simulink library "iq_mixer_8c4r_lib"  (Simulink 8.7)
settings: Solver=ode45  StartTime=0.0  StopTime=10.0  RelTol=1e-3
undefined symbols (not defined in the file): AdvDSPBChannelOutDisplay, dpoly, dspba_ChannelInVis, dspba_ChannelOutVis, dspba_internal_get_channel_ports, dspba_internal_get_demux_ports, evalAionMaskParam, latency, primtype, value
libraries: DSPBAPrim x25, Pipereg_lib x2, DSPBABase x1
settings Model: Creator=bigcat  LastModifiedBy=5g

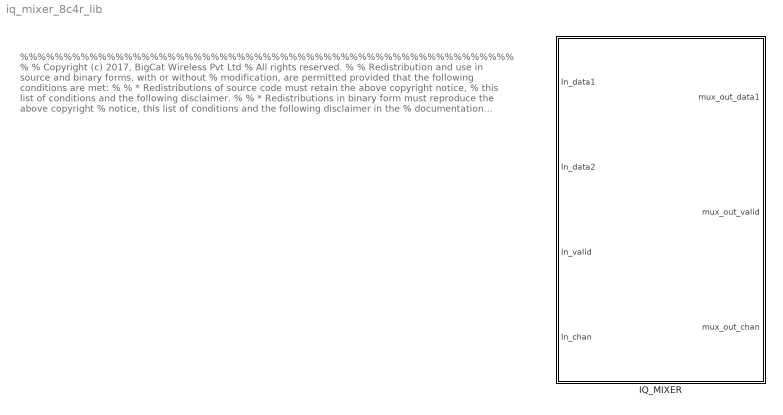
== system iq_mixer_8c4r_lib ==
  note: %%%%%%%%%%%%%%%%%%%%%%%%%%%%%%%%%%%%%%%%%%%%%%%%%%%%%%%%%
      |  %
      |  % Copyright (c) 2017, BigCat Wireless Pvt Ltd
      |  % All rights reserved.
      |  %
      |  % Redistribution and use in source and binary forms, with or without
      |  % modification, are permitted provided that the following conditions are met:
      |  %
      |  %     * Redistributions of source code must retain the above copyright notice,
      |  %       this list of conditions and the following disclaimer.
      |  %
      |  %     * Redistributions in binary form must reproduce the above copyright
      |  %       notice, this list of conditions and the following disclaimer in the
      |  %       documentation and/or other materials provided with the distribution.
      |  %
      |  %     * Neither the name of the copyright holder nor the names of its contributors
      |  %       may be used to endorse or promote products derived from this software
      |  %       without specific prior written permission.
      |  %
      |  %
      |  %
      |  % THIS SOFTWARE IS PROVIDED BY THE COPYRIGHT HOLDERS AND CONTRIBUTORS "AS IS"
      |  % AND ANY EXPRESS OR IMPLIED WARRANTIES, INCLUDING, BUT NOT LIMITED TO, THE
      |  % IMPLIED WARRANTIES OF MERCHANTABILITY AND FITNESS FOR A PARTICULAR PURPOSE ARE
      |  % DISCLAIMED. IN NO EVENT SHALL THE COPYRIGHT HOLDER OR CONTRIBUTORS BE LIABLE
      |  % FOR ANY DIRECT, INDIRECT, INCIDENTAL, SPECIAL, EXEMPLARY, OR CONSEQUENTIAL
      |  % DAMAGES (INCLUDING, BUT NOT LIMITED TO, PROCUREMENT OF SUBSTITUTE GOODS OR
      |  % SERVICES; LOSS OF USE, DATA, OR PROFITS; OR BUSINESS INTERRUPTION) HOWEVER
      |  % CAUSED AND ON ANY THEORY OF LIABILITY, WHETHER IN CONTRACT, STRICT LIABILITY,
      |  % OR TORT (INCLUDING NEGLIGENCE OR OTHERWISE) ARISING IN ANY WAY OUT OF THE USE
      |  % OF THIS SOFTWARE, EVEN IF ADVISED OF THE POSSIBILITY OF SUCH DAMAGE.
      |  %
      |   %%%%%%%%%%%%%%%%%%%%%%%%%%%%%%%%%%%%%%%%%%%%%%%%%%%%%%%%%%
  IQ_MIXER : Subsystem  mask{Latency=0, ClockMargin=0, Pipeline_stages=0}
      mask Display:
      | disp('IQ_MIXER');
      | port_label('input',1,'d_I');
      | port_label('input',2,'d_Q');
      | port_label('input',3,'v');
      | port_label('input',4,'c');
      | port_label('output',1,'q');
      | port_label('output',2,'q_v');
      | port_label('output',3,'q_c');

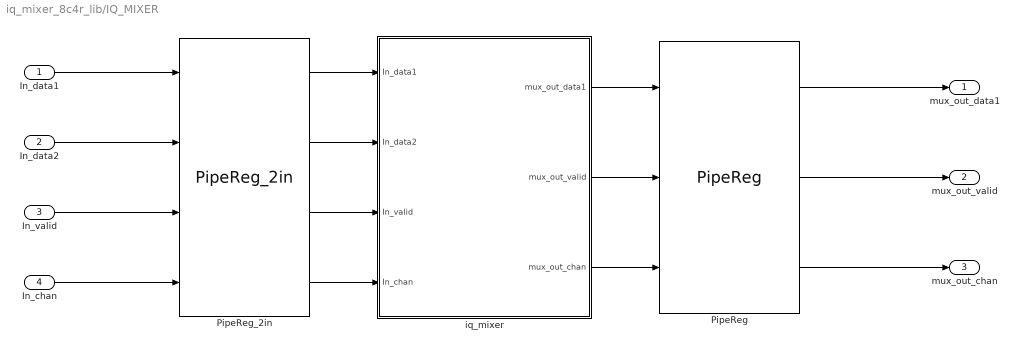
== system iq_mixer_8c4r_lib/IQ_MIXER ==
  In_data1 : Inport
  In_data2 : Inport  Port=2
  In_valid : Inport  Port=3
  In_chan : Inport  Port=4
  PipeReg : Pipereg_lib/PipeReg  NPipe=Pipeline_stages  Clock_Margin=ClockMargin
  PipeReg_2in : Pipereg_lib/PipeReg_2in  NPipe=Pipeline_stages  Clock_Margin=ClockMargin
  iq_mixer : Subsystem
  mux_out_data1 : Outport
  mux_out_valid : Outport  Port=2
  mux_out_chan : Outport  Port=3
  wires:
  PipeReg_2in/2 -> iq_mixer/2(In_data2)
  PipeReg_2in/3 -> iq_mixer/3(In_valid)
  PipeReg_2in/4 -> iq_mixer/4(In_chan)
  PipeReg_2in/1 -> iq_mixer/1(In_data1)
  iq_mixer/3(mux_out_chan) -> PipeReg/3
  iq_mixer/2(mux_out_valid) -> PipeReg/2
  iq_mixer/1(mux_out_data1) -> PipeReg/1
  In_data1/1 -> PipeReg_2in/1
  In_data2/1 -> PipeReg_2in/2
  In_valid/1 -> PipeReg_2in/3
  In_chan/1 -> PipeReg_2in/4
  PipeReg/1 -> mux_out_data1/1
  PipeReg/2 -> mux_out_valid/1
  PipeReg/3 -> mux_out_chan/1

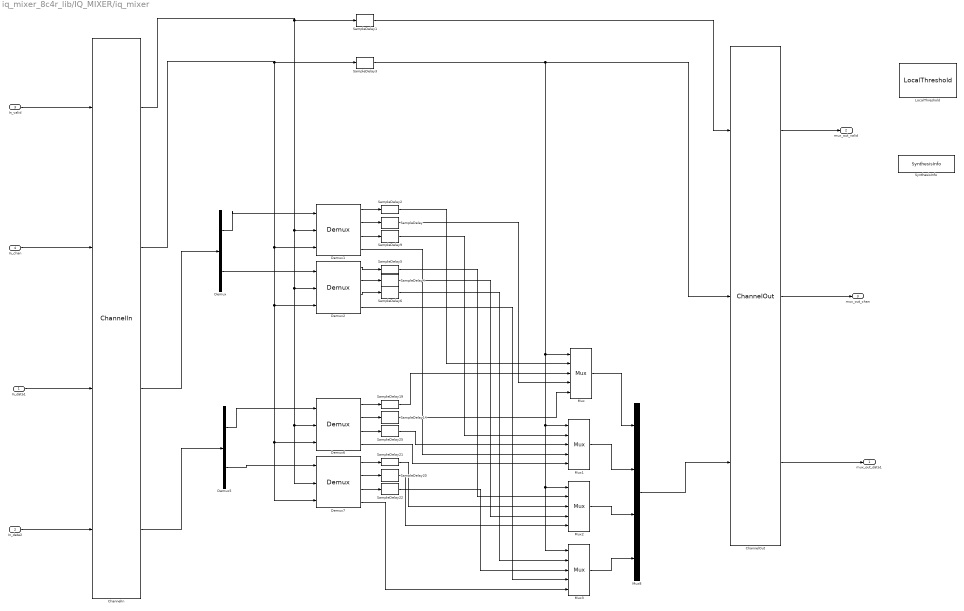
== system iq_mixer_8c4r_lib/IQ_MIXER/iq_mixer ==
  In_data1 : Inport
  In_data2 : Inport  Port=2
  In_valid : Inport  Port=3
  In_chan : Inport  Port=4
  ChannelIn : DSPBAPrim/ChannelIn  primtype=channelin  nInputs=dspba_internal_get_channel_ports(gcb)  nOutputs=dspba_internal_get_channel_ports(gcb)  omode=Inherit via internal rule  otype=sfix(16)  scale=2^-15  rndmethod=Unbiased  factor=1  satmethod=Symmetric  shift_vec=[0 1 2 -1]  value=2  inPortNames=['v'; 'c'; '0'; '1'; '2'; '3'; '4'; '5'; '6'; '7'; '8'; '9'; 'A'; 'B'; 'D'; 'E'; 'F'; 'G'; 'H'; 'I'; 'J'; 'K'; 'L'; 'M'; 'N'; 'O'; 'P'; 'Q'; 'R'; 'S'; 'T'; 'U'; 'W'; 'X'; 'Y'; 'Z']  outPortNames=['v'; 'c'; '0'; '1'; '2'; '3'; '4'; '5'; '6'; '7'; '8'; '9'; 'A'; 'B'; 'D'; 'E'; 'F'; 'G'; 'H'; 'I'; 'J'; 'K'; 'L'; 'M'; 'N'; 'O'; 'P'; 'Q'; 'R'; 'S'; 'T'; 'U'; 'W'; 'X'; 'Y'; 'Z']  dspbaimage=dspba_prim.jpg  text=fprintf('In');  style=Optimised  dataSignals=2  foldingEnabled=off  channels=1  sampleRate=200  packetBeginPresent=off  packetBeginEnabled=off  visibilities=dspba_ChannelInVis(gcb)  latencyCorrection=0  version=20141013
  ChannelOut : DSPBAPrim/ChannelOut  primtype=channelout  nInputs=dspba_internal_get_channel_ports(gcb)  nOutputs=dspba_internal_get_channel_ports(gcb)  omode=Inherit via internal rule  otype=sfix(16)  scale=2^-15  rndmethod=Unbiased  factor=1  satmethod=Symmetric  shift_vec=[0 1 2 -1]  value=1  inPortNames=['v'; 'c'; '0'; '1'; '2'; '3'; '4'; '5'; '6'; '7'; '8'; '9'; 'A'; 'B'; 'D'; 'E'; 'F'; 'G'; 'H'; 'I'; 'J'; 'K'; 'L'; 'M'; 'N'; 'O'; 'P'; 'Q'; 'R'; 'S'; 'T'; 'U'; 'W'; 'X'; 'Y'; 'Z']  outPortNames=['v'; 'c'; '0'; '1'; '2'; '3'; '4'; '5'; '6'; '7'; '8'; '9'; 'A'; 'B'; 'D'; 'E'; 'F'; 'G'; 'H'; 'I'; 'J'; 'K'; 'L'; 'M'; 'N'; 'O'; 'P'; 'Q'; 'R'; 'S'; 'T'; 'U'; 'W'; 'X'; 'Y'; 'Z']  dspbaimage=dspba_prim.jpg  text=fprintf('Out%s', AdvDSPBChannelOutDisplay(latency));  style=Optimised  dataSignals=1  foldingEnabled=off  channels=1  sampleRate=200  packetBeginPresent=off  packetBeginEnabled=off  visibilities=dspba_ChannelOutVis(gcb)  latency=41  latencyCorrection=0  version=20141013
  Demux : Demux  Outputs=2
  Demux{1..2,6..7} (4 alike) : DSPBAPrim/Demux  primtype=demux  nInputs=3  nOutputs=dspba_internal_get_demux_ports(gcb)  omode=Inherit via internal rule  otype=sfix(16)  scale=2^-15  rndmethod=Unbiased  factor=1  satmethod=Symmetric  shift_vec=[0 1 2 3]  value=4  inPortNames=['q'; 'v'; 'c']  outPortNames=['c0'; 'c1']  dspbaimage=dspba_prim.jpg  text=fprintf('demux');  style=Optimised  visibilities=1536  version=20100120
  Demux5 : Demux  Outputs=2
  LocalThreshold : DSPBABase/LocalThreshold  margin=ClockMargin  delayRegOrRAMThresholdBits=10000  MediumDualMemThresholdBits=10000  LargeDualMemThresholdBits=-1  hardMultiplierThresholdLuts=-1  version=0
  Mux{,1..3} (4 alike) : DSPBAPrim/Mux  primtype=mux  nInputs=evalAionMaskParam(gcb,'value',1)+1  nOutputs=1  omode=Inherit via internal rule  otype=sfix(16)  scale=2^-15  rndmethod=Unbiased  factor=1  satmethod=Symmetric  shift_vec=[0 1 2 -1]  value=4  inPortNames=['s'; 'd0'; 'd1'; 'd2'; 'd3'; 'd4'; 'd5'; 'd6'; 'd7'; 'd8'; 'd9';]  outPortNames=[' ']  dspbaimage=dspba_prim.jpg  text=fprintf('%s', primtype);  style=Optimised  visibilities=1032  version=20131025
  Mux8 : Mux
  SampleDelay{,4,14,20} (4 alike) : DSPBAPrim/SampleDelay  primtype=sampdelay  nInputs=1  nOutputs=1  omode=Inherit via internal rule  otype=sfix(16)  scale=2^-15  rndmethod=Unbiased  factor=1  satmethod=Symmetric  shift_vec=[0 1 2 -1]  value=2  inPortNames=[' '; ' ';]  outPortNames=[' ']  dspbaimage=dspba_prim.jpg  text=dpoly(1, eye(1,value+1), 'z')  style=Optimised  visibilities=8 + 1024 + 2^17 + 2^18  flexible=off  slackgroup=0  augmented=0  version=20090407  advOptions=[]
  SampleDelay{1..3,5,19,21} (6 alike) : DSPBAPrim/SampleDelay  primtype=sampdelay  nInputs=1  nOutputs=1  omode=Inherit via internal rule  otype=sfix(16)  scale=2^-15  rndmethod=Unbiased  factor=1  satmethod=Symmetric  shift_vec=[0 1 2 -1]  value=3  inPortNames=[' '; ' ';]  outPortNames=[' ']  dspbaimage=dspba_prim.jpg  text=dpoly(1, eye(1,value+1), 'z')  style=Optimised  visibilities=8 + 1024 + 2^17 + 2^18  flexible=off  slackgroup=0  augmented=0  version=20090407  advOptions=[]
  SampleDelay{6,9,22,25} (4 alike) : DSPBAPrim/SampleDelay  primtype=sampdelay  nInputs=1  nOutputs=1  omode=Inherit via internal rule  otype=sfix(16)  scale=2^-15  rndmethod=Unbiased  factor=1  satmethod=Symmetric  shift_vec=[0 1 2 -1]  value=1  inPortNames=[' '; ' ';]  outPortNames=[' ']  dspbaimage=dspba_prim.jpg  text=dpoly(1, eye(1,value+1), 'z')  style=Optimised  visibilities=8 + 1024 + 2^17 + 2^18  flexible=off  slackgroup=0  augmented=0  version=20090407  advOptions=[]
  SynthesisInfo : DSPBAPrim/SynthesisInfo  primtype=synthinfo  nInputs=0  nOutputs=0  omode=Inherit via internal rule  otype=sfix(16)  scale=2^-15  rndmethod=Truncate  factor=1  satmethod=Symmetric  shift_vec=[0 1 2 -1]  value=99  inPortNames=[' '; ' ';]  outPortNames=[' ']  dspbaimage=dspba_prim_ctrl.jpg  text=fprintf('Style=%s', style);  style=Scheduled  visibilities=2^15+2^17+2^18+2^19  constraintInUse=on  constraintRelation=>  constraintLimit=Latency  bitAccurate=off  version=20090407
  mux_out_data1 : Outport
  mux_out_valid : Outport  Port=2
  mux_out_chan : Outport  Port=3
  wires:
  Demux2/4 -> Mux3/4
  SampleDelay5/1 -> Mux2/2
  Mux8/1 -> ChannelOut/3
  Demux/1 -> Demux1/1
  SampleDelay25/1 -> Mux1/3
  Demux/2 -> Demux2/1
  SampleDelay14/1 -> Mux/5
  Demux5/1 -> Demux6/1
  In_valid/1 -> ChannelIn/1
  Demux6/4 -> Mux1/5
  Demux6/1 -> SampleDelay19/1
  Demux2/1 -> SampleDelay5/1
  SampleDelay9/1 -> Mux1/2
  Demux1/4 -> Mux1/4
  ChannelOut/1 -> mux_out_valid/1
  Demux7/1 -> SampleDelay21/1
  SampleDelay21/1 -> Mux2/3
  ChannelOut/2 -> mux_out_chan/1
  Demux1/2 -> SampleDelay/1
  SampleDelay4/1 -> Mux2/4
  Mux1/1 -> Mux8/2
  Demux7/2 -> SampleDelay20/1
  SampleDelay20/1 -> Mux2/5
  Demux1/3 -> SampleDelay9/1
  Demux6/2 -> SampleDelay14/1
  Demux7/3 -> SampleDelay22/1
  ChannelOut/3 -> mux_out_data1/1
  In_data1/1 -> ChannelIn/3
  Demux5/2 -> Demux7/1
  SampleDelay6/1 -> Mux3/2
  SampleDelay19/1 -> Mux/3
  Demux1/1 -> SampleDelay2/1
  ChannelIn/2 -> Demux1/3, Demux6/3, Demux7/3, Demux2/3, SampleDelay3/1
  In_data2/1 -> ChannelIn/4
  ChannelIn/4 -> Demux5/1
  SampleDelay2/1 -> Mux/2
  SampleDelay3/1 -> Mux/1, Mux1/1, Mux2/1, Mux3/1, ChannelOut/2
  Mux/1 -> Mux8/1
  Demux6/3 -> SampleDelay25/1
  Demux2/2 -> SampleDelay4/1
  Demux2/3 -> SampleDelay6/1
  SampleDelay/1 -> Mux/4
  ChannelIn/3 -> Demux/1
  SampleDelay22/1 -> Mux3/3
  In_chan/1 -> ChannelIn/2
  ChannelIn/1 -> Demux1/2, Demux2/2, Demux6/2, Demux7/2, SampleDelay1/1
  SampleDelay1/1 -> ChannelOut/1
  Demux7/4 -> Mux3/5
  Mux2/1 -> Mux8/3
  Mux3/1 -> Mux8/4
